simulink library "thc"  (R2021b)
settings: Solver=VariableStepAuto  StartTime=0.0  StopTime=10.0  RelTol=1e-3
undefined symbols (not defined in the file or in its folder): ATHC_APTCQA_X_C, ATHC_APTCQB_X_C, ATHC_dAy_X_C, ATHC_Qeq_X_kmh, ATHC_VbaseC_X_C, ATHC_VbaseC_Y_W, ATHC_VbaseD_X_C, ATHC_VbaseH_X_C, FALSE, KTHC_ACMaxMinT_sec, KTHC_aDeice_K, KTHC_AGSDefLv_K, KTHC_AGSLv1_K, KTHC_AGSLv2_K, KTHC_AGSLv3_K, KTHC_AGSLv4_K, KTHC_AGSLv5_K, KTHC_AirIntUpdateT_sec, KTHC_APTCOneZoneMax_W, KTHC_APTCPeriod_cnt, KTHC_APTCPWMEN_flg, KTHC_APTCQMaxC_W, KTHC_APTCQminC_W, KTHC_APTCQminD_W, KTHC_APTCQminRe1_W, KTHC_APTCQminRe_W, KTHC_APTCQoffT_cnt, KTHC_APTCQonT_cnt, KTHC_APTCRiLeMaxDff_W, KTHC_APTCRiLeMinDff_W, KTHC_BatInTempDef_C, KTHC_bDeice_K, KTHC_CompMaxDeice_rpm, KTHC_CompMinDeice_rpm, KTHC_CompSotxvOp_K, KTHC_CompSotxvOpLow_rpm, KTHC_CompSpdmax_rpm, KTHC_CompSpdmaxBC1_rpm, KTHC_CompSpdmaxBC_rpm, KTHC_CompSpdmid1_rpm, KTHC_CompSpdmid2_rpm, KTHC_CompSpdmid3_rpm, KTHC_CompSpdmid_rpm, KTHC_CompSpdmin_rpm, KTHC_DAPTCQ1_W, KTHC_DAPTCQ2_W, KTHC_DAPTCQ3_W, KTHC_DcChSetTemp_C, KTHC_DehumidityEN_flg, KTHC_DeiceCycTime_K, KTHC_DriveLevelWPTCBAH1_W, KTHC_DriveLevelWPTCBAH2_W, KTHC_DriveLevelWPTCBAH3_W, KTHC_DriveLevelWPTCBAH4_W, KTHC_DriveT1MinBAH_C, KTHC_DriveT2MaxBAH_C, KTHC_DriveT2MinBAH_C, KTHC_DriveT3MaxBAH_C, KTHC_DriveT3MinBAH_C, KTHC_DriveT4MaxBAH_C ... (+377)
libraries: simulink x145
(part 6 of 10)

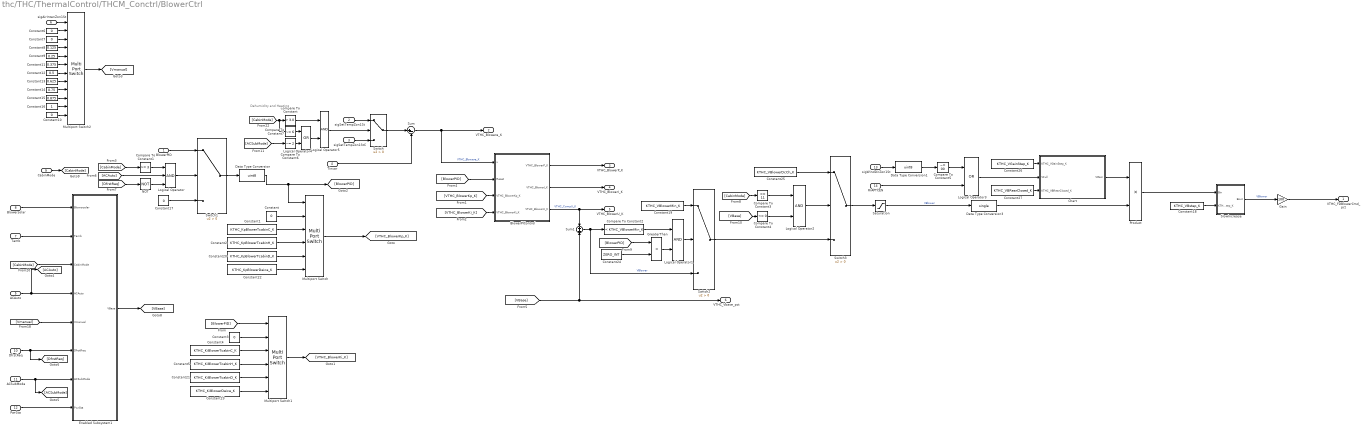
== system thc/THC/ThermalControl/THCM_Conctrl/BlowerCtrl ==
  note: Dehumidity and Heating
  BlowerPID : Inport
  sigSetTempZon1St : Inport  Port=2
  sigSetTempZon1StC : Inport  Port=3
  Tincar : Inport  Port=4
  ACAuto : Inport  Port=5
  sigAirIntenZon1St : Inport  Port=6
  Tamb : Inport  Port=7
  Blowersolar : Inport  Port=8
  CabinMode : Inport  Port=9
  DfrstReq : Inport  Port=10
  ACSubMode : Inport  Port=11
  PwrSta : Inport  Port=12
  sigWindDirZon1St : Inport  Port=13
  RrAPTCEN : Inport  Port=14
  BlowerPIControl : Subsystem
  Chart : Stateflow chart  TreatAsAtomicUnit=on
      settings: PortSchema="{\"entries\":[{\"content\":{\"sides\":[{\"content\":{\"connectorIds\":[\"In3\",\"In1\",\"In2\"]},\"type\":\"ConnectorPlacement.EquallySpacedRectSide\",\"uuid\":\"ac038b54-0c63-4b1e-9440-2050b36ef882\"},{\"content\":{\"connectorIds\":[\"Out1\"],\"side\":\"RIGHT\"},\"type\":\"ConnectorPlacement.EquallySpacedRectSide\",\"uuid\":\"d3d16d57-d9ad-415c-8d7c-688e16dd7c1f\"},{\"content\":{\"connectorIds\":[],\"side\":\"TOP\"},\"type\":\"ConnectorPlacement.EquallySpacedRectSide\",\"uuid\":\"ce9b93c1-3cd7-4e15-ac68-a22916c5a1d9\"}]},\"type\":\"ConnectorPlacement.EquallySpacedConnector\",\"uuid\":\"5542f07e-e2fc-49c6-8325-c7b19e9c9c98\"}],\"packageUris\":[\"http://schema.mathworks.com/mf0/Connector/R2020b\"],\"version\":\"1.0\"}"
  Compare To Constant : simulink/Logic and Bit Operations/Compare To Constant  relop=>  const=3.0  OutDataTypeStr=boolean
  Compare To Constant1 : simulink/Logic and Bit Operations/Compare To Constant  relop=>=  const=3  OutDataTypeStr=boolean
  Compare To Constant2 : simulink/Logic and Bit Operations/Compare To Constant  relop=<  const=KTHC_VBlowerMin_K  OutDataTypeStr=boolean
  Compare To Constant3 : simulink/Logic and Bit Operations/Compare To Constant  relop===  const=11  OutDataTypeStr=boolean
  Compare To Constant4 : simulink/Logic and Bit Operations/Compare To Constant  relop=<=  const=0  OutDataTypeStr=boolean
  Compare To Constant5 : simulink/Logic and Bit Operations/Compare To Constant  relop=~=  const=00  OutDataTypeStr=boolean
  Compare To Constant6 : simulink/Logic and Bit Operations/Compare To Constant  relop=~=  const=2  OutDataTypeStr=boolean
  Compare To Constant7 : simulink/Logic and Bit Operations/Compare To Constant  relop=~=  const=6  OutDataTypeStr=boolean
  Constant{,3,6..7,10,17} (6 alike) : Constant  Value=0
  Constant1 : Constant  Value=KTHC_KpBlowerTcabinC_K
  Constant11 : Constant  Value=0.375
  Constant12 : Constant  Value=0.5
  Constant13 : Constant  Value=0.625
  Constant14 : Constant  Value=0.75
  Constant15 : Constant  Value=0.875
  Constant16 : Constant
  Constant18 : Constant  Value=KTHC_VBstep_K
  Constant19 : Constant  Value=KTHC_VBlowerMin_K
  Constant2 : Constant  Value=KTHC_KpBlowerTcabinH_K
  Constant20 : Constant  Value=KTHC_KpBlowerTcabinD_K
  Constant21 : Constant  Value=KTHC_KiBlowerTcabinD_K
  Constant22 : Constant  Value=KTHC_KpBlowerDeice_K
  Constant23 : Constant  Value=KTHC_KiBlowerDeice_K
  Constant24 : Constant  Value=ZERO_INT
  Constant25 : Constant  Value=KTHC_VBlowerDcCh_K
  Constant26 : Constant  Value=KTHC_VGainStep_K
  Constant27 : Constant  Value=KTHC_VBRearClosed_K
  Constant4 : Constant  Value=KTHC_KiBlowerTcabinC_K
  Constant5 : Constant  Value=KTHC_KiBlowerTcabinH_K
  Constant8 : Constant  Value=0.125
  Constant9 : Constant  Value=0.25
  Data Type Conversion : DataTypeConversion  OutDataTypeStr=uint8
  Data Type Conversion1 : DataTypeConversion  OutDataTypeStr=uint8
  Data Type Conversion3 : DataTypeConversion  OutDataTypeStr=single
  Enabled Subsystem1 : Subsystem  TreatAsAtomicUnit=on
  Gain : Gain  Gain=100
  GreaterThan : RelationalOperator  Operator=>  OutDataTypeStr=boolean  RndMeth=Simplest
  Logical Operator : Logic  Inputs=3  AllPortsSameDT=off  OutDataTypeStr=boolean
  Logical Operator1 : Logic  AllPortsSameDT=off  OutDataTypeStr=boolean
  Logical Operator2 : Logic  AllPortsSameDT=off  OutDataTypeStr=boolean
  Logical Operator3 : Logic  Operator=OR  AllPortsSameDT=off  OutDataTypeStr=boolean
  Logical Operator4 : Logic  Operator=OR  AllPortsSameDT=off  OutDataTypeStr=boolean
  Logical Operator5 : Logic  AllPortsSameDT=off  OutDataTypeStr=boolean
  Multiport Switch : MultiPortSwitch  DataPortOrder=Zero-based contiguous  Inputs=5  zeroidx=on
  Multiport Switch1 : MultiPortSwitch  DataPortOrder=Zero-based contiguous  Inputs=5  zeroidx=on
  Multiport Switch2 : MultiPortSwitch  DataPortOrder=Zero-based contiguous  Inputs=11  zeroidx=on
  NOT : Logic  Operator=NOT  IconShape=distinctive  AllPortsSameDT=off  OutDataTypeStr=boolean
  Product : Product
  Saturation : Saturate  UpperLimit=1  LowerLimit=0
  SlowIncrease : Stateflow chart  TreatAsAtomicUnit=on
  Sum : Sum  Inputs=|+-
  Sum1 : Sum  Inputs=+|+
  Switch{,1..3} (4 alike) : Switch  Criteria=u2 > Threshold
  VTHC_FDBlowerCmd_pct : Outport
  VTHC_Blowere_K : Outport  Port=2
  VTHC_BlowerP_K : Outport  Port=3
  VTHC_BlowerI_K : Outport  Port=4
  VTHC_BlowerU_K : Outport  Port=5
  VTHC_Vbase_pct : Outport  Port=6
  wires:
  [VBase] -> Compare To Constant4/1
  Compare To Constant4/1 -> Logical Operator2/2
  Compare To Constant3/1 -> Logical Operator2/1
  Logical Operator2/1 -> Switch3/2
  Constant25/1 -> Switch3/1
  [CabinMode] -> Compare To Constant3/1
  Switch3/1 -> Saturation/1
  Switch2/1 -> Switch3/3
  GreaterThan/1 -> Logical Operator1/2
  Constant24/1 -> GreaterThan/2
  Switch1/1 -> Data Type Conversion/1
  Constant23/1 -> Multiport Switch1/6
  Constant22/1 -> Multiport Switch/6
  Constant19/1 -> Switch2/1
  Logical Operator1/1 -> Switch2/2
  Compare To Constant2/1 -> Logical Operator1/1
  [BlowerPID] -> GreaterThan/1
  Constant18/1 -> SlowIncrease/2(KTHC_VBstep_K)
  Saturation/1 -> Data Type Conversion3/1  "VBlower"
  PwrSta/1 -> Enabled Subsystem1/8(PwrSta)
  NOT/1 -> Logical Operator/3
  [DfrstReq] -> NOT/1
  [ACAuto] -> Logical Operator/2
  Logical Operator/1 -> Switch1/2
  Constant17/1 -> Switch1/3
  [CabinMode] -> Compare To Constant1/1
  Compare To Constant1/1 -> Logical Operator/1
  BlowerPID/1 -> Switch1/1
  SlowIncrease/1(Bout) -> Gain/1  "VBlower"
  Constant21/1 -> Multiport Switch1/5
  Constant20/1 -> Multiport Switch/5
  Compare To Constant/1 -> Logical Operator5/1
  [CabinMode] -> Compare To Constant7/1, Compare To Constant/1
  [CabinMode] -> Enabled Subsystem1/3(CabinMode)
  DfrstReq/1 -> Enabled Subsystem1/6(DfrstReq), [DfrstReq]
  Gain/1 -> VTHC_FDBlowerCmd_pct/1
  Constant5/1 -> Multiport Switch1/4
  Constant1/1 -> Multiport Switch/3
  Enabled Subsystem1/1(VBase) -> [VBase]
  Constant6/1 -> Multiport Switch2/2
  [VTHC_BlowerKi_K] -> BlowerPIControl/4(VTHC_BlowerKi_K)
  BlowerPIControl/3(VTHC_BlowerU_K) -> Sum1/1, VTHC_BlowerU_K/1  "VTHC_CompU_K"
  Constant2/1 -> Multiport Switch/4
  Constant10/1 -> Multiport Switch2/12
  [BlowerPID] -> BlowerPIControl/2(Reset)
  Multiport Switch1/1 -> [VTHC_BlowerKi_K]
  sigSetTempZon1StC/1 -> Switch/3
  [BlowerPID] -> Multiport Switch1/1
  Constant/1 -> Multiport Switch/2
  Constant3/1 -> Multiport Switch1/2
  Data Type Conversion/1 -> [BlowerPID], Multiport Switch/1
  Constant11/1 -> Multiport Switch2/6
  BlowerPIControl/1(VTHC_BlowerP_K) -> VTHC_BlowerP_K/1
  Tincar/1 -> Sum/2
  Constant16/1 -> Multiport Switch2/11
  Constant4/1 -> Multiport Switch1/3
  Constant13/1 -> Multiport Switch2/8
  sigSetTempZon1St/1 -> Switch/1
  [VBase] -> Sum1/2, VTHC_Vbase_pct/1
  Sum1/1 -> Switch2/3, Compare To Constant2/1  "VBlower"
  Sum/1 -> BlowerPIControl/1(x), VTHC_Blowere_K/1  "VTHC_Blowere_K"
  Constant8/1 -> Multiport Switch2/4
  [VTHC_BlowerKp_K] -> BlowerPIControl/3(VTHC_BlowerKp_K)
  BlowerPIControl/2(VTHC_BlowerI_K) -> VTHC_BlowerI_K/1
  ACAuto/1 -> Enabled Subsystem1/4(ACAuto), [ACAuto]
  Switch/1 -> Sum/1
  Multiport Switch/1 -> [VTHC_BlowerKp_K]
  [Vmanual] -> Enabled Subsystem1/5(Vmanual)
  sigAirIntenZon1St/1 -> Multiport Switch2/1
  Constant15/1 -> Multiport Switch2/10
  Constant14/1 -> Multiport Switch2/9
  Constant9/1 -> Multiport Switch2/5
  Constant7/1 -> Multiport Switch2/3
  Constant12/1 -> Multiport Switch2/7
  Blowersolar/1 -> Enabled Subsystem1/1(Blowersolar)
  Multiport Switch2/1 -> [Vmanual]
  Tamb/1 -> Enabled Subsystem1/2(Tamb)
  CabinMode/1 -> [CabinMode]
  sigWindDirZon1St/1 -> Data Type Conversion1/1
  RrAPTCEN/1 -> Logical Operator3/2
  Data Type Conversion1/1 -> Compare To Constant5/1
  Compare To Constant5/1 -> Logical Operator3/1
  Logical Operator3/1 -> Chart/1(VFull)
  Constant26/1 -> Chart/3(KTHC_VGainStep_K)
  Constant27/1 -> Chart/2(KTHC_VBRearClosed_K)
  Chart/1(VGain) -> Product/1
  Data Type Conversion3/1 -> Product/2
  Product/1 -> SlowIncrease/1(Bin)
  ACSubMode/1 -> [ACSubMode], Enabled Subsystem1/7(ACSubMode)
  [ACSubMode] -> Compare To Constant6/1
  Compare To Constant7/1 -> Logical Operator4/1
  Compare To Constant6/1 -> Logical Operator4/2
  Logical Operator4/1 -> Logical Operator5/2
  Logical Operator5/1 -> Switch/2

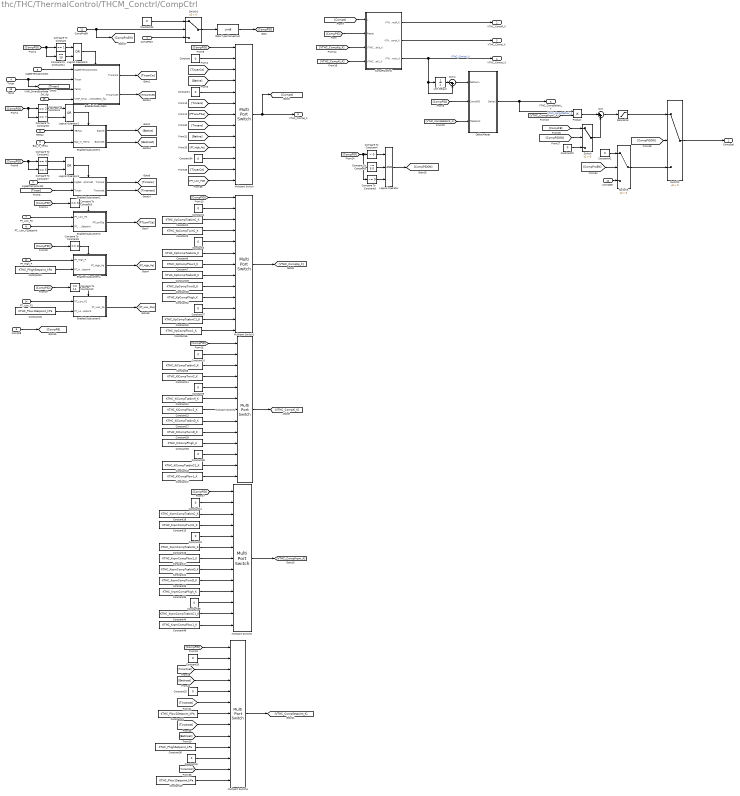
== system thc/THC/ThermalControl/THCM_Conctrl/CompCtrl ==
  CompPIDin : Inport
  sigSetTempZon1St : Inport  Port=2
  sigSetTempZon1StC : Inport  Port=3
  Tincar : Inport  Port=4
  TBMax : Inport  Port=5
  Bat_In_Temp : Inport  Port=6
  PT_Low_P2 : Inport  Port=7
  PT_ Low_P2Setpoint : Inport  Port=8
  CompFB : Inport  Port=9
  CompSet : Inport  Port=10
  CompProEN : Inport  Port=11
  PT_High_P : Inport  Port=12
  Tamb : Inport  Port=13
  PT_Low_P1 : Inport  Port=14
  VINP_SmartEcoModeSW_flg : Inport  Port=15
  CompPIControl : Subsystem
  Compare To Constant : simulink/Logic and Bit Operations/Compare To Constant  relop===  const=1  OutDataTypeStr=boolean
  Compare To Constant1 : simulink/Logic and Bit Operations/Compare To Constant  relop===  const=2  OutDataTypeStr=boolean
  Compare To Constant10 : simulink/Logic and Bit Operations/Compare To Constant  relop===  const=11  OutDataTypeStr=boolean
  Compare To Constant11 : simulink/Logic and Bit Operations/Compare To Constant  relop===  const=10  OutDataTypeStr=boolean
  Compare To Constant2 : simulink/Logic and Bit Operations/Compare To Constant  relop===  const=4  OutDataTypeStr=boolean
  Compare To Constant3 : simulink/Logic and Bit Operations/Compare To Constant  relop===  const=5  OutDataTypeStr=boolean
  Compare To Constant4 : simulink/Logic and Bit Operations/Compare To Constant  relop=>  const=0  OutDataTypeStr=boolean
  Compare To Constant5 : simulink/Logic and Bit Operations/Compare To Constant  relop=~=  const=3.0  OutDataTypeStr=boolean
  Compare To Constant6 : simulink/Logic and Bit Operations/Compare To Constant  relop===  const=7  OutDataTypeStr=boolean
  Compare To Constant7 : simulink/Logic and Bit Operations/Compare To Constant  relop===  const=6  OutDataTypeStr=boolean
  Compare To Constant8 : simulink/Logic and Bit Operations/Compare To Constant  relop===  const=8  OutDataTypeStr=boolean
  Compare To Constant9 : simulink/Logic and Bit Operations/Compare To Constant  relop=~=  const=9  OutDataTypeStr=boolean
  Constant{,1,3..4,9..10,14,19..20,22..23,25,34,37..41} (18 alike) : Constant  Value=0
  Constant11 : Constant  Value=KTHC_KiCompTwinC_K
  Constant12 : Constant  Value=KTHC_KiCompTcabinH_K
  Constant13 : Constant  Value=KTHC_KiCompPlow2_K
  Constant15 : Constant  Value=KTHC_KrpmCompTwinC_K
  Constant16 : Constant  Value=KTHC_KrpmCompTcabinH_K
  Constant17 : Constant  Value=KTHC_KrpmCompPlow2_K
  Constant18 : Constant  Value=KTHC_KrpmCompTcabinC_K
  Constant2 : Constant  Value=KTHC_KpCompTcabinC_K
  Constant21 : Constant  Value=KTHC_Plow2Setpoint_kPa
  Constant24 : Constant  Value=KTHC_KrpmCompTcabinD_K
  Constant26 : Constant  Value=KTHC_KrpmCompTwinD_K
  Constant27 : Constant  Value=KTHC_KiCompTcabinD_K
  Constant28 : Constant  Value=KTHC_KiCompTwinD_K
  Constant29 : Constant  Value=KTHC_KpCompTcabinD_K
  Constant30 : Constant  Value=KTHC_KpCompTwinD_K
  Constant31 : Constant  Value=KTHC_PhighSetpoint_kPa
  Constant32 : Constant  Value=KTHC_KpCompPhigh_K
  Constant33 : Constant  Value=KTHC_KiCompPhigh_K
  Constant35 : Constant  Value=KTHC_KrpmCompPhigh_K
  Constant36 : Constant  Value=KTHC_PhighSetpoint_kPa
  Constant42 : Constant  Value=KTHC_KpCompTcabinC1_K
  Constant43 : Constant  Value=KTHC_KiCompTcabinC1_K
  Constant44 : Constant  Value=KTHC_KrpmCompTcabinC1_K
  Constant45 : Constant  Value=KTHC_Plow1Setpoint_kPa
  Constant46 : Constant  Value=KTHC_KpCompPlow1_K
  Constant47 : Constant  Value=KTHC_KiCompPlow1_K
  Constant48 : Constant  Value=KTHC_KrpmCompPlow1_K
  Constant49 : Constant  Value=KTHC_Plow1Setpoint_kPa
  Constant5 : Constant  Value=KTHC_KpCompTwinC_K
  Constant6 : Constant  Value=KTHC_KpCompTcabinH_K
  Constant7 : Constant  Value=KTHC_KpCompPlow2_K
  Constant8 : Constant  Value=KTHC_KiCompTcabinC_K
  Data Type Conversion : DataTypeConversion  OutDataTypeStr=uint8
  DeltaUReset : Subsystem
  Enabled Subsystem : Subsystem  TreatAsAtomicUnit=on
  Enabled Subsystem1 : Subsystem  TreatAsAtomicUnit=on
  Enabled Subsystem2 : Subsystem  TreatAsAtomicUnit=on
  Enabled Subsystem3 : Subsystem  TreatAsAtomicUnit=on
  Enabled Subsystem4 : Subsystem  TreatAsAtomicUnit=on
  Enabled Subsystem5 : Subsystem  TreatAsAtomicUnit=on
  Logical Operator : Logic  Inputs=3  AllPortsSameDT=off  OutDataTypeStr=boolean
  Logical Operator1 : Logic  Operator=OR  AllPortsSameDT=off  OutDataTypeStr=boolean
  Logical Operator2 : Logic  Operator=OR  AllPortsSameDT=off  OutDataTypeStr=boolean
  Logical Operator3 : Logic  Operator=OR  AllPortsSameDT=off  OutDataTypeStr=boolean
  Multiport Switch{,1..4} (5 alike) : MultiPortSwitch  DataPortOrder=Zero-based contiguous  Inputs=12  DiagnosticForDefault=None  zeroidx=on
  Product : Product
  Saturation : Saturate  UpperLimit=KTHC_CompSpdmax_rpm  LowerLimit=KTHC_CompSpdmin_rpm  OutDataTypeStr=double
  Sum : Sum  Inputs=|++
  Sum4 : Sum  Inputs=|-+
  Switch{,1..3} (4 alike) : Switch  Criteria=u2 > Threshold
  Unit Delay2 : UnitDelay  SampleTime=-1  HasFrameUpgradeWarning=on
  CompSpd : Outport
  VTHC_CompP_K : Outport  Port=2
  VTHC_CompI_K : Outport  Port=3
  VTHC_CompU_K : Outport  Port=4
  VTHC_CompDeltaU_K : Outport  Port=5
  VTHC_Compe_K : Outport  Port=6
  wires:
  VINP_SmartEcoModeSW_flg/1 -> Enabled Subsystem/4(VINP_SmartEcoModeSW_flg)
  Compare To Constant11/1 -> Logical Operator3/2
  Logical Operator3/1 -> Enabled Subsystem/Enable
  Constant49/1 -> Multiport Switch4/13
  Constant48/1 -> Multiport Switch3/13
  Constant47/1 -> Multiport Switch2/13
  Constant46/1 -> Multiport Switch1/13
  [PT_Low_P1e] -> Multiport Switch/13
  Enabled Subsystem5/1(PT_Low_Pe) -> [PT_Low_P1e]
  PT_Low_P1/1 -> Enabled Subsystem5/1(PT_Low_P1)
  Compare To Constant10/1 -> Enabled Subsystem5/Enable
  [CompPID] -> Compare To Constant10/1
  Constant45/1 -> Enabled Subsystem5/2(PT_Low_P1Setpoint)
  [TincarCset] -> Multiport Switch4/12
  Constant44/1 -> Multiport Switch3/12
  Constant43/1 -> Multiport Switch2/12
  Constant42/1 -> Multiport Switch1/12
  [TincarCe] -> Multiport Switch/12
  Data Type Conversion/1 -> [CompPID]
  Tamb/1 -> Enabled Subsystem/3(Tamb)
  [CompProEN] -> Switch3/2
  Constant41/1 -> Switch3/1
  Switch3/1 -> Switch2/3
  Constant40/1 -> Multiport Switch4/11
  Compare To Constant9/1 -> Logical Operator/3
  Constant39/1 -> Multiport Switch3/11
  Constant38/1 -> Multiport Switch2/11
  Constant37/1 -> Multiport Switch1/11
  Constant34/1 -> Multiport Switch/11
  Constant35/1 -> Multiport Switch3/10
  Constant36/1 -> Multiport Switch4/10
  Constant33/1 -> Multiport Switch2/10
  Constant32/1 -> Multiport Switch1/10
  [PT_High_Pe] -> Multiport Switch/10
  Constant31/1 -> Enabled Subsystem4/2(PT_High_PSetpoint)
  [CompPID] -> Compare To Constant8/1
  Compare To Constant8/1 -> Enabled Subsystem4/Enable
  PT_High_P/1 -> Enabled Subsystem4/1(PT_High_P)
  Enabled Subsystem4/1(PT_High_Pe) -> [PT_High_Pe]
  [BatIne] -> Multiport Switch/9
  [Tincare] -> Multiport Switch/8
  Constant30/1 -> Multiport Switch1/9
  Constant29/1 -> Multiport Switch1/8
  Constant28/1 -> Multiport Switch2/9
  Constant27/1 -> Multiport Switch2/8
  Constant26/1 -> Multiport Switch3/9
  Constant24/1 -> Multiport Switch3/8
  [BatInset] -> Multiport Switch4/9
  [Tincarset] -> Multiport Switch4/8
  Compare To Constant2/1 -> Logical Operator2/1
  [CompPID] -> Compare To Constant7/1, Compare To Constant2/1
  Compare To Constant7/1 -> Logical Operator2/2
  Logical Operator2/1 -> Enabled Subsystem2/Enable
  Logical Operator1/1 -> Enabled Subsystem1/Enable
  Compare To Constant6/1 -> Logical Operator1/2
  Switch1/1 -> Data Type Conversion/1
  Constant23/1 -> Switch1/1
  CompProEN/1 -> Switch1/2, [CompProEN]
  [CompPID] -> Multiport Switch/1
  [TincarCset] -> Multiport Switch4/3
  CompPIDin/1 -> Switch1/3
  [Tincare] -> Multiport Switch/6
  Constant11/1 -> Multiport Switch2/4
  CompPIControl/1(VTHC_CompP_K) -> VTHC_CompP_K/1
  Enabled Subsystem1/1(BatIne) -> [BatIne]
  Enabled Subsystem/2(TincarCset) -> [TincarCset]
  [CompFB] -> Switch/1
  [PTLowP2e] -> Multiport Switch/7
  Enabled Subsystem/1(TincarCe) -> [TincarCe]
  Constant15/1 -> Multiport Switch3/4
  Enabled Subsystem3/1(PTLowP2e) -> [PTLowP2e]
  PT_Low_P2/1 -> Enabled Subsystem3/1(PT_Low_P2)
  Constant6/1 -> Multiport Switch1/6
  Enabled Subsystem2/1(Tincare) -> [Tincare]
  Constant21/1 -> Multiport Switch4/7
  Multiport Switch1/1 -> [VTHC_CompKp_K]
  [CompPID] -> Multiport Switch1/1
  DeltaUReset/1(DeltaU) -> Product/1, VTHC_CompDeltaU_K/1  "VTHC_CompDeltaU_K"
  [CompPID] -> Multiport Switch3/1
  CompPIControl/3(VTHC_CompU_K) -> VTHC_CompU_K/1, Unit Delay2/1, Sum4/2  "VTHC_CompU_K"
  CompSet/1 -> Switch3/3
  Constant19/1 -> Multiport Switch3/5
  [CompPID] -> Compare To Constant/1, Compare To Constant11/1
  Constant18/1 -> Multiport Switch3/3
  TBMax/1 -> Enabled Subsystem1/1(TBMax)
  Multiport Switch3/1 -> [VTHC_CompKrpm_K]
  [VTHC_CompKi_K] -> CompPIControl/4(VTHC_CompKi_K)
  Constant16/1 -> Multiport Switch3/6
  Sum4/1 -> DeltaUReset/1(DeltaUin)
  Constant17/1 -> Multiport Switch3/7
  Constant14/1 -> Multiport Switch3/2
  [CompPIDON] -> Switch/2
  Compare To Constant5/1 -> Logical Operator/2
  sigSetTempZon1StC/1 -> Enabled Subsystem/1(sigSetTempZon1StC)
  Constant4/1 -> Multiport Switch1/2
  Logical Operator/1 -> [CompPIDON]
  Compare To Constant4/1 -> Logical Operator/1
  [VTHC_CompSetpoint_K] -> DeltaUReset/3(TSetpoint)
  CompPIControl/2(VTHC_CompI_K) -> VTHC_CompI_K/1
  [CompPIDON] -> Switch2/2
  [CompPID] -> Compare To Constant1/1, Compare To Constant6/1
  Compare To Constant/1 -> Logical Operator3/1
  [VTHC_CompKrpm_K] -> Product/2
  Saturation/1 -> Switch2/1
  Sum/1 -> Saturation/1
  Multiport Switch/1 -> VTHC_Compe_K/1, [Compe]
  [Tincarset] -> Multiport Switch4/6
  Switch2/1 -> CompSpd/1
  [Tincar] -> Enabled Subsystem2/2(Tincar)
  Compare To Constant3/1 -> Enabled Subsystem3/Enable
  [CompPID] -> CompPIControl/2(Reset)
  [TincarCe] -> Multiport Switch/3
  Tincar/1 -> Enabled Subsystem/2(Tincar), [Tincar]
  Constant/1 -> Multiport Switch/2
  [CompPID] -> Compare To Constant3/1
  [CompPID] -> DeltaUReset/2(CompPID)
  Unit Delay2/1 -> Sum4/1
  Bat_In_Temp/1 -> Enabled Subsystem1/2(Bat_In_Temp)
  Constant8/1 -> Multiport Switch2/3
  Constant2/1 -> Multiport Switch1/3
  [VTHC_CompKp_K] -> CompPIControl/3(VTHC_CompKp_K)
  Enabled Subsystem2/2(Tincarset) -> [Tincarset]
  Enabled Subsystem1/2(BatInset) -> [BatInset]
  Product/1 -> Sum/1
  [BatIne] -> Multiport Switch/4
  CompFB/1 -> [CompFB]
  [Compe] -> CompPIControl/1(x)
  Compare To Constant1/1 -> Logical Operator1/1
  Constant1/1 -> Multiport Switch/5
  Constant3/1 -> Multiport Switch1/5
  sigSetTempZon1St/1 -> Enabled Subsystem2/1(sigSetTempZon1St)
  [BatInset] -> Multiport Switch4/4
  PT_ Low_P2Setpoint/1 -> Enabled Subsystem3/2(PT_ Low_P2Setpoint)
  Constant7/1 -> Multiport Switch1/7
  Constant5/1 -> Multiport Switch1/4
  Constant10/1 -> Multiport Switch2/2
  Constant13/1 -> Multiport Switch2/7
  Multiport Switch2/1 -> [VTHC_CompKi_K]
  Constant9/1 -> Multiport Switch2/5
  [CompPID] -> Multiport Switch2/1
  Constant12/1 -> Multiport Switch2/6
  Constant20/1 -> Multiport Switch4/2
  Constant25/1 -> Multiport Switch4/5
  [CompPID] -> Multiport Switch4/1
  Multiport Switch4/1 -> [VTHC_CompSetpoint_K]
  Switch/1 -> Sum/2
  Constant22/1 -> Switch/3
  [CompPID] -> Compare To Constant4/1, Compare To Constant5/1, Compare To Constant9/1

== system thc/THC/ThermalControl/THCM_Conctrl/EWP1 ==
  EWPLV : Inport
  Constant : Constant  Value=KTHC_EWPLv1_K
  Constant1 : Constant  Value=KTHC_EWPLv2_K
  Constant2 : Constant  Value=KTHC_EWPLv3_K
  Constant3 : Constant  Value=KTHC_EWPLv4_K
  Constant4 : Constant  Value=KTHC_EWPLv5_K
  Constant5 : Constant  Value=0
  Constant6 : Constant  Value=KTHC_EWP3SpdDeice_K
  Constant7 : Constant  Value=125
  Constant8 : Constant  Value=KTHC_EWPDcCharge_K
  Multiport Switch : MultiPortSwitch  Inputs=9  DiagnosticForDefault=None
  EWPOut : Outport
  wires:
  Constant8/1 -> Multiport Switch/9
  Constant6/1 -> Multiport Switch/7
  Multiport Switch/1 -> EWPOut/1
  Constant2/1 -> Multiport Switch/4
  Constant1/1 -> Multiport Switch/3
  Constant/1 -> Multiport Switch/2
  Constant3/1 -> Multiport Switch/5
  Constant4/1 -> Multiport Switch/6
  Constant5/1 -> Multiport Switch/10
  EWPLV/1 -> Multiport Switch/1
  Constant7/1 -> Multiport Switch/8

== system thc/THC/ThermalControl/THCM_Conctrl/EWP2 ==
  EWPLV : Inport
  Constant : Constant  Value=KTHC_EWPLv1_K
  Constant1 : Constant  Value=KTHC_EWPLv2_K
  Constant2 : Constant  Value=KTHC_EWPLv3_K
  Constant3 : Constant  Value=KTHC_EWPLv4_K
  Constant4 : Constant  Value=KTHC_EWPLv5_K
  Constant5 : Constant  Value=0
  Constant6 : Constant  Value=KTHC_EWP3SpdDeice_K
  Constant7 : Constant  Value=125
  Constant8 : Constant  Value=KTHC_EWPDcCharge_K
  Multiport Switch : MultiPortSwitch  Inputs=9  DiagnosticForDefault=None
  EWPOut : Outport
  wires:
  Constant7/1 -> Multiport Switch/8
  EWPLV/1 -> Multiport Switch/1
  Constant5/1 -> Multiport Switch/10
  Constant4/1 -> Multiport Switch/6
  Constant3/1 -> Multiport Switch/5
  Constant/1 -> Multiport Switch/2
  Constant1/1 -> Multiport Switch/3
  Constant2/1 -> Multiport Switch/4
  Multiport Switch/1 -> EWPOut/1
  Constant6/1 -> Multiport Switch/7
  Constant8/1 -> Multiport Switch/9

== system thc/THC/ThermalControl/THCM_Conctrl/EWP3 ==
  EWPLV : Inport
  Constant : Constant  Value=KTHC_EWPLv1_K
  Constant1 : Constant  Value=KTHC_EWPLv2_K
  Constant2 : Constant  Value=KTHC_EWPLv3_K
  Constant3 : Constant  Value=KTHC_EWPLv4_K
  Constant4 : Constant  Value=KTHC_EWPLv5_K
  Constant5 : Constant  Value=0
  Constant6 : Constant  Value=KTHC_EWP3SpdDeice_K
  Constant7 : Constant  Value=125
  Constant8 : Constant  Value=KTHC_EWPDcCharge_K
  Multiport Switch : MultiPortSwitch  Inputs=9  DiagnosticForDefault=None
  EWPOut : Outport
  wires:
  Constant7/1 -> Multiport Switch/8
  EWPLV/1 -> Multiport Switch/1
  Constant5/1 -> Multiport Switch/10
  Constant4/1 -> Multiport Switch/6
  Constant3/1 -> Multiport Switch/5
  Constant/1 -> Multiport Switch/2
  Constant1/1 -> Multiport Switch/3
  Constant2/1 -> Multiport Switch/4
  Multiport Switch/1 -> EWPOut/1
  Constant6/1 -> Multiport Switch/7
  Constant8/1 -> Multiport Switch/9

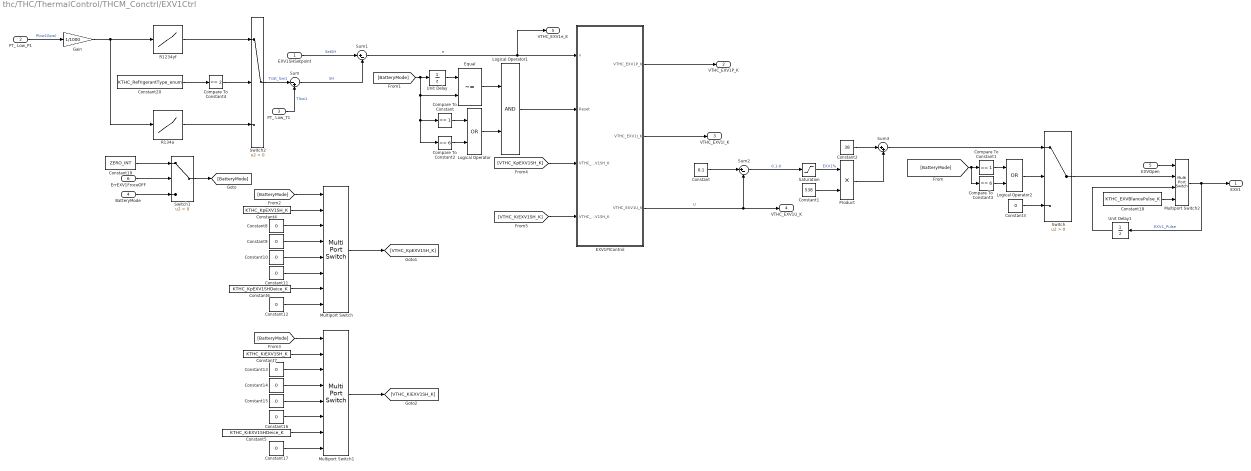
== system thc/THC/ThermalControl/THCM_Conctrl/EXV1Ctrl ==
  EXV1SHSetpoint : Inport
  PT_ Low_P1 : Inport  Port=2
  PT_ Low_T1 : Inport  Port=3
  BatteryMode : Inport  Port=4
  EXVOpen : Inport  Port=5
  ErrEXV1FroceOFF : Inport  Port=6
  Compare To Constant : simulink/Logic and Bit Operations/Compare To Constant  relop===  const=1  OutDataTypeStr=boolean
  Compare To Constant1 : simulink/Logic and Bit Operations/Compare To Constant  relop===  const=1  OutDataTypeStr=boolean
  Compare To Constant2 : simulink/Logic and Bit Operations/Compare To Constant  relop===  const=6  OutDataTypeStr=boolean
  Compare To Constant3 : simulink/Logic and Bit Operations/Compare To Constant  relop===  const=6  OutDataTypeStr=boolean
  Compare To Constant4 : simulink/Logic and Bit Operations/Compare To Constant  relop===  const=2  OutDataTypeStr=boolean
  Constant : Constant  Value=0.1
  Constant1 : Constant  Value=538
  Constant{3,8..17} (11 alike) : Constant  Value=0
  Constant18 : Constant  Value=KTHC_EXVBlancePulse_K
  Constant19 : Constant  Value=ZERO_INT
  Constant2 : Constant  Value=38
  Constant20 : Constant  Value=KTHC_RefrigerantType_enum
  Constant4 : Constant  Value=KTHC_KpEXV1SH_K
  Constant5 : Constant  Value=KTHC_KiEXV1SHDeice_K
  Constant6 : Constant  Value=KTHC_KpEXV1SHDeice_K
  Constant7 : Constant  Value=KTHC_KiEXV1SH_K
  EXV1PIControl : Subsystem
  Equal : RelationalOperator  Operator=~=  OutDataTypeStr=boolean  RndMeth=Simplest
  Gain : Gain  Gain=1/1000
  Logical Operator : Logic  Operator=OR  AllPortsSameDT=off  OutDataTypeStr=boolean
  Logical Operator1 : Logic  AllPortsSameDT=off  OutDataTypeStr=boolean
  Logical Operator2 : Logic  Operator=OR  AllPortsSameDT=off  OutDataTypeStr=boolean
  Multiport Switch : MultiPortSwitch  Inputs=7  DiagnosticForDefault=None
  Multiport Switch1 : MultiPortSwitch  Inputs=7  DiagnosticForDefault=None
  Multiport Switch2 : MultiPortSwitch  DataPortOrder=Zero-based contiguous  zeroidx=on
  Product : Product
  R1234yf : Lookup_n-D  NumberOfTableDimensions=1  BreakpointsForDimension1=[0.03742 0.06237 0.09906 0.11778 0.15092 0.1909 0.2386 0.29495 0.36092 0.43753 0.52583 0.6269 0.74189 0.87197 1.0184 1.3023]  Table=[-50 -40 -30 -26 -20 -14 -8 -2 4 10 16 22 28 34 40 50]  InternalRulePriority=Speed  RndMeth=Simplest  InputSameDT=on
  R134a : Lookup_n-D  NumberOfTableDimensions=1  BreakpointsForDimension1=[0.02945 0.05121 0.08438 0.10167 0.13273 0.17082 0.21693 0.27217 0.33766 0.41461 0.50425 0.60789 0.72688 0.86263 1.0166 1.31790]  Table=[-50 -40 -30 -26 -20 -14 -8 -2 4 10 16 22 28 34 40 50]  InternalRulePriority=Speed  RndMeth=Simplest  InputSameDT=on
  Saturation : Saturate  UpperLimit=1  LowerLimit=0
  Sum : Sum  Inputs=|-+
  Sum1 : Sum  Inputs=|+-
  Sum2 : Sum  Inputs=|+-
  Sum3 : Sum  Inputs=|++
  Switch : Switch  Criteria=u2 > Threshold
  Switch1 : Switch  Criteria=u2 > Threshold
  Switch2 : Switch  Criteria=u2 > Threshold
  Unit Delay : UnitDelay  SampleTime=-1  HasFrameUpgradeWarning=on
  Unit Delay1 : UnitDelay  SampleTime=-1  HasFrameUpgradeWarning=on
  EXV1 : Outport
  VTHC_EXV1P_K : Outport  Port=2
  VTHC_EXV1I_K : Outport  Port=3
  VTHC_EXV1U_K : Outport  Port=4
  VTHC_EXV1e_K : Outport  Port=5
  wires:
  Constant20/1 -> Compare To Constant4/1
  R134a/1 -> Switch2/3
  Gain/1 -> R134a/1, R1234yf/1
  Compare To Constant4/1 -> Switch2/2
  R1234yf/1 -> Switch2/1
  BatteryMode/1 -> Switch1/3
  Switch1/1 -> [BatteryMode]
  ErrEXV1FroceOFF/1 -> Switch1/2
  Constant19/1 -> Switch1/1
  Unit Delay1/1 -> Multiport Switch2/3
  EXVOpen/1 -> Multiport Switch2/1
  Constant18/1 -> Multiport Switch2/4
  Switch/1 -> Multiport Switch2/2
  [VTHC_KiEXV1SH_K] -> EXV1PIControl/4(VTHC_KiEXV1SH_K)
  Multiport Switch1/1 -> [VTHC_KiEXV1SH_K]
  [VTHC_KpEXV1SH_K] -> EXV1PIControl/3(VTHC_KpEXV1SH_K)
  Multiport Switch/1 -> [VTHC_KpEXV1SH_K]
  Constant17/1 -> Multiport Switch1/8
  Constant16/1 -> Multiport Switch1/6
  Constant15/1 -> Multiport Switch1/5
  Constant14/1 -> Multiport Switch1/4
  Constant13/1 -> Multiport Switch1/3
  Constant12/1 -> Multiport Switch/8
  Constant11/1 -> Multiport Switch/6
  Constant10/1 -> Multiport Switch/5
  Constant9/1 -> Multiport Switch/4
  Constant8/1 -> Multiport Switch/3
  [BatteryMode] -> Multiport Switch1/1
  Constant7/1 -> Multiport Switch1/2
  Constant5/1 -> Multiport Switch1/7
  Constant6/1 -> Multiport Switch/7
  Constant4/1 -> Multiport Switch/2
  [BatteryMode] -> Multiport Switch/1
  Logical Operator2/1 -> Switch/2
  Compare To Constant3/1 -> Logical Operator2/2
  Compare To Constant1/1 -> Logical Operator2/1
  Logical Operator1/1 -> EXV1PIControl/2(Reset)
  Logical Operator/1 -> Logical Operator1/2
  Equal/1 -> Logical Operator1/1
  Compare To Constant2/1 -> Logical Operator/2
  Compare To Constant/1 -> Logical Operator/1
  Unit Delay/1 -> Equal/1
  [BatteryMode] -> Equal/2, Compare To Constant2/1, Compare To Constant/1, Unit Delay/1
  EXV1PIControl/2(VTHC_EXV1I_K) -> VTHC_EXV1I_K/1
  EXV1PIControl/1(VTHC_EXV1P_K) -> VTHC_EXV1P_K/1
  PT_ Low_T1/1 -> Sum/2  "Tlow1"
  Sum2/1 -> Saturation/1  "0.1-U"
  Constant2/1 -> Sum3/1
  Constant/1 -> Sum2/1
  Product/1 -> Sum3/2
  Saturation/1 -> Product/1  "EXV1%"
  Switch2/1 -> Sum/1  "Tsat_low1"
  EXV1SHSetpoint/1 -> Sum1/1  "SetSH"
  Multiport Switch2/1 -> EXV1/1, Unit Delay1/1  "EXV1_Pulse"
  EXV1PIControl/3(VTHC_EXV1U_K) -> Sum2/2, VTHC_EXV1U_K/1  "U"
  Sum/1 -> Sum1/2  "SH"
  PT_ Low_P1/1 -> Gain/1  "Plow1(kpa)"
  Constant3/1 -> Switch/3
  [BatteryMode] -> Compare To Constant1/1, Compare To Constant3/1
  Constant1/1 -> Product/2
  Sum1/1 -> EXV1PIControl/1(x), VTHC_EXV1e_K/1  "e"
  Sum3/1 -> Switch/1

== system thc/THC/ThermalControl/THCM_Conctrl/EXV2Ctrl ==
  EXV2SHSetpoint : Inport
  PT_ Low_T2 : Inport  Port=2
  PT_ Low_P2 : Inport  Port=3
  EXV2PIDMode : Inport  Port=4
  EXVOpen : Inport  Port=5
  ErrEXV2FroceOFF : Inport  Port=6
  Compare To Constant : simulink/Logic and Bit Operations/Compare To Constant  relop=>  const=0  OutDataTypeStr=boolean
  Compare To Constant1 : simulink/Logic and Bit Operations/Compare To Constant  relop===  const=2  OutDataTypeStr=boolean
  Constant : Constant  Value=0.1
  Constant1 : Constant  Value=538
  Constant10 : Constant  Value=KTHC_EXVBlancePulse_K
  Constant11 : Constant  Value=ZERO_INT
  Constant12 : Constant  Value=KTHC_RefrigerantType_enum
  Constant2 : Constant  Value=38
  Constant3 : Constant  Value=0
  Constant4 : Constant  Value=0
  Constant5 : Constant  Value=KTHC_KpEXV2SH_K
  Constant6 : Constant  Value=KTHC_KiEXV2SH_K
  Constant7 : Constant  Value=0
  Constant8 : Constant  Value=KTHC_KpEXV2SHD_K
  Constant9 : Constant  Value=KTHC_KiEXV2SHD_K
  EXV2PIControl : Subsystem
  Gain : Gain  Gain=1/1000
  Multiport Switch : MultiPortSwitch  DataPortOrder=Zero-based contiguous  zeroidx=on
  Multiport Switch1 : MultiPortSwitch  DataPortOrder=Zero-based contiguous  zeroidx=on
  Multiport Switch2 : MultiPortSwitch  DataPortOrder=Zero-based contiguous  zeroidx=on
  Product : Product
  R1234yf : Lookup_n-D  NumberOfTableDimensions=1  BreakpointsForDimension1=[0.03742 0.06237 0.09906 0.11778 0.15092 0.1909 0.2386 0.29495 0.36092 0.43753 0.52583 0.6269 0.74189 0.87197 1.0184 1.3023]  Table=[-50 -40 -30 -26 -20 -14 -8 -2 4 10 16 22 28 34 40 50]  InternalRulePriority=Speed  RndMeth=Simplest  InputSameDT=on
  R134a : Lookup_n-D  NumberOfTableDimensions=1  BreakpointsForDimension1=[0.02945 0.05121 0.08438 0.10167 0.13273 0.17082 0.21693 0.27217 0.33766 0.41461 0.50425 0.60789 0.72688 0.86263 1.0166 1.31790]  Table=[-50 -40 -30 -26 -20 -14 -8 -2 4 10 16 22 28 34 40 50]  InternalRulePriority=Speed  RndMeth=Simplest  InputSameDT=on
  Saturation3 : Saturate  UpperLimit=1  LowerLimit=0
  Sum10 : Sum  Inputs=|++
  Sum7 : Sum  Inputs=|-+
  Sum8 : Sum  Inputs=|+-
  Sum9 : Sum  Inputs=|-+
  Switch : Switch  Criteria=u2 > Threshold
  Switch1 : Switch  Criteria=u2 > Threshold
  Switch2 : Switch  Criteria=u2 > Threshold
  Unit Delay1 : UnitDelay  SampleTime=-1  HasFrameUpgradeWarning=on
  EXV2 : Outport
  Tsat_low2 : Outport  Port=2
  VTHC_EXV2P_K : Outport  Port=3
  VTHC_EXV2I_K : Outport  Port=4
  VTHC_EXV2U_K : Outport  Port=5
  VTHC_EXV2e_K : Outport  Port=6
  wires:
  R134a/1 -> Switch2/3
  Compare To Constant1/1 -> Switch2/2
  Constant12/1 -> Compare To Constant1/1
  R1234yf/1 -> Switch2/1
  Switch1/1 -> [EXV2PIDMode]
  Constant11/1 -> Switch1/1
  ErrEXV2FroceOFF/1 -> Switch1/2
  Switch/1 -> Multiport Switch2/2
  Constant10/1 -> Multiport Switch2/4
  EXVOpen/1 -> Multiport Switch2/1
  Unit Delay1/1 -> Multiport Switch2/3
  Multiport Switch2/1 -> EXV2/1, Unit Delay1/1  "EXV2_Pulse"
  Constant3/1 -> Switch/3
  Compare To Constant/1 -> Switch/2
  [EXV2PIDMode] -> Compare To Constant/1
  [KiEXV2] -> EXV2PIControl/4(VTHC_KiEXV2_K)
  Constant9/1 -> Multiport Switch1/4
  Constant6/1 -> Multiport Switch1/3
  Multiport Switch1/1 -> [KiEXV2]
  [KpEXV2] -> EXV2PIControl/3(VTHC_KpEXV2_K)
  Constant8/1 -> Multiport Switch/4
  Constant5/1 -> Multiport Switch/3
  Multiport Switch/1 -> [KpEXV2]
  [EXV2PIDMode] -> Multiport Switch1/1
  Constant7/1 -> Multiport Switch1/2
  Constant4/1 -> Multiport Switch/2
  [EXV2PIDMode] -> Multiport Switch/1
  [EXV2PIDMode] -> EXV2PIControl/2(Reset)
  EXV2PIControl/2(VTHC_EXV2I_K) -> VTHC_EXV2I_K/1
  EXV2PIControl/1(VTHC_EXV2P_K) -> VTHC_EXV2P_K/1
  Product/1 -> Sum10/2
  Sum8/1 -> EXV2PIControl/1(x), VTHC_EXV2e_K/1  "e"
  Switch2/1 -> Sum7/1, Tsat_low2/1  "Tsat_low2"
  EXV2SHSetpoint/1 -> Sum8/1
  PT_ Low_P2/1 -> Gain/1
  EXV2PIDMode/1 -> Switch1/3
  Sum10/1 -> Switch/1  "EXV2_Pulse"
  PT_ Low_T2/1 -> Sum7/2  "Tlow2"
  Sum7/1 -> Sum8/2  "SH"
  Constant2/1 -> Sum10/1
  Saturation3/1 -> Product/1  "EXV2%"
  Gain/1 -> R134a/1, R1234yf/1
  Sum9/1 -> Saturation3/1  "0.1-U"
  Constant1/1 -> Product/2
  Constant/1 -> Sum9/2
  EXV2PIControl/3(VTHC_EXV2U_K) -> Sum9/1, VTHC_EXV2U_K/1  "U"

== system thc/THC/ThermalControl/THCM_Conctrl/RadiatorFan ==
  FAN : Inport
  AGS_Err : Inport  Port=2
  AGS : Inport  Port=3
  Compare To Constant : simulink/Logic and Bit Operations/Compare To Constant  relop=>  const=1  OutDataTypeStr=boolean
  Constant : Constant  Value=KTHC_FANLv1_pct
  Constant1 : Constant  Value=KTHC_FANLv2_pct
  Constant2 : Constant  Value=KTHC_FANLv3_pct
  Constant3 : Constant  Value=KTHC_FANLv4_pct
  Constant4 : Constant  Value=KTHC_FANLv5_pct
  Constant5 : Constant  Value=0
  Constant6 : Constant  Value=KTHC_FANDefLv_pct
  Constant7 : Constant  Value=KTHC_ErrHandleEN_flg
  Logical Operator : Logic  Inputs=3  AllPortsSameDT=off  OutDataTypeStr=boolean
  Multiport Switch : MultiPortSwitch  Inputs=6  DiagnosticForDefault=None
  Switch : Switch  Criteria=u2 > Threshold
  CoolgFanActDuty : Outport
  wires:
  Constant7/1 -> Logical Operator/3
  Multiport Switch/1 -> Switch/3
  Switch/1 -> CoolgFanActDuty/1
  Compare To Constant/1 -> Logical Operator/2
  AGS_Err/1 -> Logical Operator/1
  AGS/1 -> Compare To Constant/1
  Constant6/1 -> Switch/1
  Logical Operator/1 -> Switch/2
  Constant3/1 -> Multiport Switch/5
  Constant2/1 -> Multiport Switch/4
  Constant1/1 -> Multiport Switch/3
  Constant4/1 -> Multiport Switch/6
  Constant5/1 -> Multiport Switch/7
  Constant/1 -> Multiport Switch/2
  FAN/1 -> Multiport Switch/1

== system thc/THC/ThermalControl/THCM_Conctrl/SensorErrorHandle1 ==
  DataIn : Inport
  SensorError : Inport  Port=2
  PresetValue : Inport  Port=3
  Constant : Constant  Value=KTHC_ErrHandleEN_flg
  Logical Operator : Logic  AllPortsSameDT=off  OutDataTypeStr=boolean
  Switch : Switch  Criteria=u2 > Threshold
  DataOut : Outport
  wires:
  Constant/1 -> Logical Operator/2
  SensorError/1 -> Logical Operator/1
  Logical Operator/1 -> Switch/2
  Switch/1 -> DataOut/1
  DataIn/1 -> Switch/3
  PresetValue/1 -> Switch/1

== system thc/THC/ThermalControl/THCM_Conctrl/SensorErrorHandle10 ==
  DataIn : Inport
  SensorError : Inport  Port=2
  PresetValue : Inport  Port=3
  Constant : Constant  Value=KTHC_ErrHandleEN_flg
  Logical Operator : Logic  AllPortsSameDT=off  OutDataTypeStr=boolean
  Switch : Switch  Criteria=u2 > Threshold
  DataOut : Outport
  wires:
  PresetValue/1 -> Switch/1
  DataIn/1 -> Switch/3
  Switch/1 -> DataOut/1
  Logical Operator/1 -> Switch/2
  SensorError/1 -> Logical Operator/1
  Constant/1 -> Logical Operator/2

== system thc/THC/ThermalControl/THCM_Conctrl/SensorErrorHandle11 ==
  DataIn : Inport
  SensorError : Inport  Port=2
  PresetValue : Inport  Port=3
  Constant : Constant  Value=KTHC_ErrHandleEN_flg
  Logical Operator : Logic  AllPortsSameDT=off  OutDataTypeStr=boolean
  Switch : Switch  Criteria=u2 > Threshold
  DataOut : Outport
  wires:
  PresetValue/1 -> Switch/1
  DataIn/1 -> Switch/3
  Switch/1 -> DataOut/1
  Logical Operator/1 -> Switch/2
  SensorError/1 -> Logical Operator/1
  Constant/1 -> Logical Operator/2

== system thc/THC/ThermalControl/THCM_Conctrl/SensorErrorHandle12 ==
  DataIn : Inport
  SensorError : Inport  Port=2
  PresetValue : Inport  Port=3
  Constant : Constant  Value=KTHC_ErrHandleEN_flg
  Logical Operator : Logic  AllPortsSameDT=off  OutDataTypeStr=boolean
  Switch : Switch  Criteria=u2 > Threshold
  DataOut : Outport
  wires:
  PresetValue/1 -> Switch/1
  DataIn/1 -> Switch/3
  Switch/1 -> DataOut/1
  Logical Operator/1 -> Switch/2
  SensorError/1 -> Logical Operator/1
  Constant/1 -> Logical Operator/2

== system thc/THC/ThermalControl/THCM_Conctrl/SensorErrorHandle2 ==
  DataIn : Inport
  SensorError : Inport  Port=2
  PresetValue : Inport  Port=3
  Constant : Constant  Value=KTHC_ErrHandleEN_flg
  Logical Operator : Logic  AllPortsSameDT=off  OutDataTypeStr=boolean
  Switch : Switch  Criteria=u2 > Threshold
  DataOut : Outport
  wires:
  PresetValue/1 -> Switch/1
  DataIn/1 -> Switch/3
  Switch/1 -> DataOut/1
  Logical Operator/1 -> Switch/2
  SensorError/1 -> Logical Operator/1
  Constant/1 -> Logical Operator/2

== system thc/THC/ThermalControl/THCM_Conctrl/SensorErrorHandle3 ==
  DataIn : Inport
  SensorError : Inport  Port=2
  PresetValue : Inport  Port=3
  Constant : Constant  Value=KTHC_ErrHandleEN_flg
  Logical Operator : Logic  AllPortsSameDT=off  OutDataTypeStr=boolean
  Switch : Switch  Criteria=u2 > Threshold
  DataOut : Outport
  wires:
  Constant/1 -> Logical Operator/2
  SensorError/1 -> Logical Operator/1
  Logical Operator/1 -> Switch/2
  Switch/1 -> DataOut/1
  DataIn/1 -> Switch/3
  PresetValue/1 -> Switch/1

== system thc/THC/ThermalControl/THCM_Conctrl/SensorErrorHandle4 ==
  DataIn : Inport
  SensorError : Inport  Port=2
  PresetValue : Inport  Port=3
  Constant : Constant  Value=KTHC_TevaErrHandleEN_flg
  Logical Operator : Logic  AllPortsSameDT=off  OutDataTypeStr=boolean
  Switch : Switch  Criteria=u2 > Threshold
  DataOut : Outport
  wires:
  Constant/1 -> Logical Operator/2
  SensorError/1 -> Logical Operator/1
  Logical Operator/1 -> Switch/2
  Switch/1 -> DataOut/1
  DataIn/1 -> Switch/3
  PresetValue/1 -> Switch/1

== system thc/THC/ThermalControl/THCM_Conctrl/SensorErrorHandle5 ==
  DataIn : Inport
  SensorError : Inport  Port=2
  PresetValue : Inport  Port=3
  Constant : Constant  Value=KTHC_TevaErrHandleEN_flg
  Logical Operator : Logic  AllPortsSameDT=off  OutDataTypeStr=boolean
  Switch : Switch  Criteria=u2 > Threshold
  DataOut : Outport
  wires:
  PresetValue/1 -> Switch/1
  DataIn/1 -> Switch/3
  Switch/1 -> DataOut/1
  Logical Operator/1 -> Switch/2
  SensorError/1 -> Logical Operator/1
  Constant/1 -> Logical Operator/2

== system thc/THC/ThermalControl/THCM_Conctrl/SensorErrorHandle6 ==
  DataIn : Inport
  SensorError : Inport  Port=2
  PresetValue : Inport  Port=3
  Constant : Constant  Value=KTHC_TevaErrHandleEN_flg
  Logical Operator : Logic  AllPortsSameDT=off  OutDataTypeStr=boolean
  Switch : Switch  Criteria=u2 > Threshold
  DataOut : Outport
  wires:
  Constant/1 -> Logical Operator/2
  SensorError/1 -> Logical Operator/1
  Logical Operator/1 -> Switch/2
  Switch/1 -> DataOut/1
  DataIn/1 -> Switch/3
  PresetValue/1 -> Switch/1

== system thc/THC/ThermalControl/THCM_Conctrl/SensorErrorHandle7 ==
  DataIn : Inport
  SensorError : Inport  Port=2
  PresetValue : Inport  Port=3
  Constant : Constant  Value=KTHC_TevaErrHandleEN_flg
  Logical Operator : Logic  AllPortsSameDT=off  OutDataTypeStr=boolean
  Switch : Switch  Criteria=u2 > Threshold
  DataOut : Outport
  wires:
  PresetValue/1 -> Switch/1
  DataIn/1 -> Switch/3
  Switch/1 -> DataOut/1
  Logical Operator/1 -> Switch/2
  SensorError/1 -> Logical Operator/1
  Constant/1 -> Logical Operator/2

== system thc/THC/ThermalControl/THCM_Conctrl/SensorErrorHandle8 ==
  DataIn : Inport
  SensorError : Inport  Port=2
  PresetValue : Inport  Port=3
  Constant : Constant  Value=KTHC_TevaErrHandleEN_flg
  Logical Operator : Logic  AllPortsSameDT=off  OutDataTypeStr=boolean
  Switch : Switch  Criteria=u2 > Threshold
  DataOut : Outport
  wires:
  Constant/1 -> Logical Operator/2
  SensorError/1 -> Logical Operator/1
  Logical Operator/1 -> Switch/2
  Switch/1 -> DataOut/1
  DataIn/1 -> Switch/3
  PresetValue/1 -> Switch/1

== system thc/THC/ThermalControl/THCM_Conctrl/SensorErrorHandle9 ==
  DataIn : Inport
  SensorError : Inport  Port=2
  PresetValue : Inport  Port=3
  Constant : Constant  Value=KTHC_TevaErrHandleEN_flg
  Logical Operator : Logic  AllPortsSameDT=off  OutDataTypeStr=boolean
  Switch : Switch  Criteria=u2 > Threshold
  DataOut : Outport
  wires:
  PresetValue/1 -> Switch/1
  DataIn/1 -> Switch/3
  Switch/1 -> DataOut/1
  Logical Operator/1 -> Switch/2
  SensorError/1 -> Logical Operator/1
  Constant/1 -> Logical Operator/2

== system thc/THC/ThermalControl/THCM_Conctrl/Subsystem ==
  CompSpd : Inport
  CabinMode : Inport  Port=2
  CompFB : Inport  Port=3
  Chart : Stateflow chart  TreatAsAtomicUnit=on
      settings: PortSchema="{\"entries\":[{\"content\":{\"sides\":[{\"content\":{\"connectorIds\":[\"In7\",\"In1\",\"In2\",\"In3\",\"In4\",\"In5\",\"In6\",\"In8\",\"In9\",\"In10\",\"In11\"]},\"type\":\"ConnectorPlacement.EquallySpacedRectSide\",\"uuid\":\"1db6d48d-2993-4fd1-a317-039acf53791d\"},{\"content\":{\"connectorIds\":[\"Out1\",\"Out2\",\"Out3\"],\"side\":\"RIGHT\"},\"type\":\"ConnectorPlacement.EquallySpacedRectSide\",\"uuid\":\"3b07bc2c-8788-4d9a-bac7-12ac97bb3dfe\"},{\"content\":{\"connectorIds\":[],\"side\":\"TOP\"},\"type\":\"ConnectorPlacement.EquallySpacedRectSide\",\"uuid\":\"678ef0de-745c-42f5-bb8c-af17f8a0632e\"}]},\"type\":\"ConnectorPlacement.EquallySpacedConnector\",\"uuid\":\"729d42ab-7bc1-4f80-88b9-90079b8c4930\"}],\"packageUris\":[\"http://schema.mathworks.com/mf0/Connector/R2020b\"],\"version\":\"1.0\"}"
  Compare To Constant : simulink/Logic and Bit Operations/Compare To Constant  relop=>=  const=2  OutDataTypeStr=boolean
  Compare To Constant1 : simulink/Logic and Bit Operations/Compare To Constant  relop=>  const=3  OutDataTypeStr=boolean
  Compare To Constant10 : simulink/Logic and Bit Operations/Compare To Constant  relop=<  const=10  OutDataTypeStr=boolean
  Compare To Constant11 : simulink/Logic and Bit Operations/Compare To Constant  relop===  const=9  OutDataTypeStr=boolean
  Compare To Constant12 : simulink/Logic and Bit Operations/Compare To Constant  relop===  const=1  OutDataTypeStr=boolean
  Compare To Constant13 : simulink/Logic and Bit Operations/Compare To Constant  relop===  const=5  OutDataTypeStr=boolean
  Compare To Constant2 : simulink/Logic and Bit Operations/Compare To Constant  relop=>=  const=1  OutDataTypeStr=boolean
  Compare To Constant3 : simulink/Logic and Bit Operations/Compare To Constant  relop=<=  const=3  OutDataTypeStr=boolean
  Compare To Constant4 : simulink/Logic and Bit Operations/Compare To Constant  relop===  const=8  OutDataTypeStr=boolean
  Compare To Constant5 : simulink/Logic and Bit Operations/Compare To Constant  relop===  const=6  OutDataTypeStr=boolean
  Compare To Constant6 : simulink/Logic and Bit Operations/Compare To Constant  relop===  const=7  OutDataTypeStr=boolean
  Compare To Constant7 : simulink/Logic and Bit Operations/Compare To Constant  relop===  const=4  OutDataTypeStr=boolean
  Compare To Constant8 : simulink/Logic and Bit Operations/Compare To Constant  relop=~=  const=7  OutDataTypeStr=boolean
  Compare To Constant9 : simulink/Logic and Bit Operations/Compare To Constant  relop=>=  const=10  OutDataTypeStr=boolean
  Constant3 : Constant  Value=0
  Constant4 : Constant  Value=KTHC_PBlaceTime1_K
  Constant5 : Constant  Value=KTHC_PBlaceTime2_K
  Constant6 : Constant  Value=KTHC_PBlaceTime3_K
  Constant7 : Constant  Value=KTHC_PBlaceTime4_K
  Logical Operator : Logic  AllPortsSameDT=off  OutDataTypeStr=boolean
  Logical Operator1 : Logic  Operator=OR  Inputs=4  AllPortsSameDT=off  OutDataTypeStr=boolean
  Logical Operator2 : Logic  Operator=OR  Inputs=4  AllPortsSameDT=off  OutDataTypeStr=boolean
  Logical Operator3 : Logic  Operator=OR  AllPortsSameDT=off  OutDataTypeStr=boolean
  Logical Operator4 : Logic  Inputs=3  AllPortsSameDT=off  OutDataTypeStr=boolean
  Logical Operator7 : Logic  Operator=NOT  AllPortsSameDT=off  OutDataTypeStr=boolean
  Logical Operator8 : Logic  AllPortsSameDT=off  OutDataTypeStr=boolean
  NOT : Logic  Operator=NOT  IconShape=distinctive  AllPortsSameDT=off  OutDataTypeStr=boolean
  NOT1 : Logic  Operator=NOT  IconShape=distinctive  AllPortsSameDT=off  OutDataTypeStr=boolean
  NOT2 : Logic  Operator=NOT  IconShape=distinctive  AllPortsSameDT=off  OutDataTypeStr=boolean
  Switch{,2,4,6} (4 alike) : Switch  Criteria=u2 > Threshold
  Unit Delay{,1..5} (6 alike) : UnitDelay  SampleTime=-1  HasFrameUpgradeWarning=on
  FD_Comp_Cmd : Outport
  FD_SOV1_Cmd : Outport  Port=2
  FD_SOV2_Cmd : Outport  Port=3
  FD_SOV3_Cmd : Outport  Port=4
  EXVOpen : Outport  Port=5
  wires:
  Compare To Constant4/1 -> Logical Operator2/1
  Compare To Constant11/1 -> Logical Operator2/2
  Constant7/1 -> Chart/11(KTHC_PBlaceTime4_K)
  Chart/3(EXVOpen) -> EXVOpen/1
  Constant6/1 -> Chart/10(KTHC_PBlaceTime3_K)
  Constant5/1 -> Chart/9(KTHC_PBlaceTime2_K)
  Constant4/1 -> Chart/8(KTHC_PBlaceTime1_K)
  Compare To Constant13/1 -> Logical Operator2/4
  Compare To Constant10/1 -> Logical Operator4/3
  Compare To Constant9/1 -> Logical Operator1/4
  Compare To Constant8/1 -> Logical Operator4/2
  Logical Operator4/1 -> Logical Operator3/2
  Compare To Constant7/1 -> Logical Operator2/3
  CabinMode/1 -> Compare To Constant3/1, Compare To Constant2/1, Compare To Constant/1, Compare To Constant6/1, Compare To Constant12/1, Compare To Constant1/1, Compare To Constant8/1, Compare To Constant10/1, Compare To Constant4/1, Compare To Constant13/1, Compare To Constant7/1, Compare To Constant11/1, Compare To Constant9/1, Compare To Constant5/1
  Compare To Constant6/1 -> Logical Operator1/3
  Compare To Constant5/1 -> Logical Operator1/2
  Logical Operator/1 -> Logical Operator1/1
  Compare To Constant/1 -> Logical Operator8/1
  CompFB/1 -> Chart/7(Comp)
  Compare To Constant1/1 -> Logical Operator4/1
  Compare To Constant2/1 -> Logical Operator/1
  Compare To Constant3/1 -> Logical Operator/2
  Compare To Constant12/1 -> Logical Operator3/1
  Chart/1(FCompOFF) -> Logical Operator7/1
  Logical Operator8/1 -> Switch6/2
  Constant3/1 -> Switch6/3
  Switch6/1 -> FD_Comp_Cmd/1  "FD_Comp_Cmd"
  CompSpd/1 -> Switch6/1
  Logical Operator7/1 -> Logical Operator8/2
  NOT2/1 -> FD_SOV3_Cmd/1  "FD_SOV3_Cmd"
  NOT1/1 -> FD_SOV2_Cmd/1  "FD_SOV2_Cmd"
  NOT/1 -> FD_SOV1_Cmd/1  "FD_SOV1_Cmd"
  [Keep] -> Switch4/2
  [SOV3C] -> Switch4/3
  Switch4/1 -> NOT2/1, Unit Delay5/1
  Unit Delay5/1 -> Switch4/1
  Unit Delay4/1 -> Switch2/1
  Switch2/1 -> NOT1/1, Unit Delay4/1
  [SOV2C] -> Switch2/3
  [Keep] -> Switch2/2
  [Keep] -> Switch/2
  [SOV1C] -> Switch/3
  Chart/2(Keep) -> [Keep]
  Switch/1 -> NOT/1, Unit Delay3/1
  Unit Delay3/1 -> Switch/1
  Unit Delay2/1 -> Chart/6(SOV3CBuf)
  Logical Operator2/1 -> Unit Delay2/1, Chart/5(SOV3C), [SOV3C]
  Logical Operator3/1 -> Chart/3(SOV2C), [SOV2C], Unit Delay1/1
  Unit Delay1/1 -> Chart/4(SOV2CBuf)
  Unit Delay/1 -> Chart/2(SOV1CBuf)
  Logical Operator1/1 -> Chart/1(SOV1C), [SOV1C], Unit Delay/1
